simulink model "Task12"  (R2022b)
settings: Solver=VariableStepAuto  StartTime=0.0  StopTime=10.0  RelTol=1e-3
settings Model: Creator=LOQ  LastModifiedBy=LOQ
settings OptimizationCC: ReuseModelBlockBuffer=on
settings RTWCC: GPUComputeCapability=5.0
settings ConfigComp: CovBoundaryAbsTol=1.0e-5

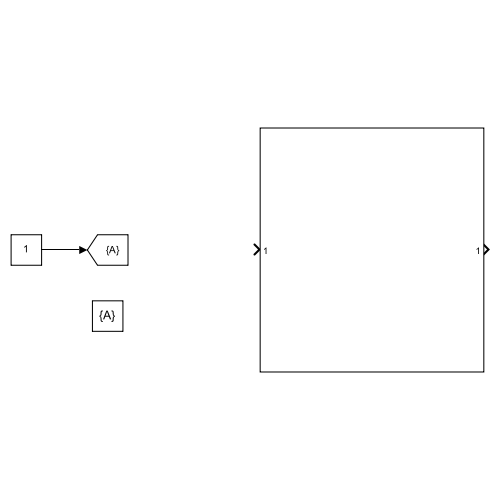
[thumbnail: Simulink's stored preview of the top-level diagram]
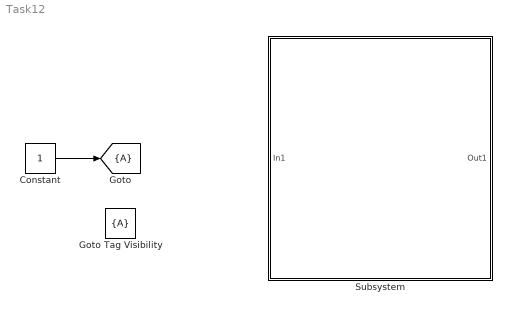
== system Task12 ==
  Constant : Constant
  Goto : Goto  TagVisibility=scoped
  Goto Tag Visibility : GotoTagVisibility
  Subsystem : Subsystem
  wires:
  Constant/1 -> Goto/1

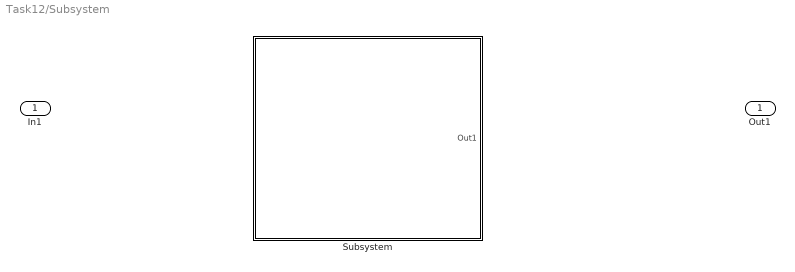
== system Task12/Subsystem ==
  In1 : Inport
  Subsystem : Subsystem
  Out1 : Outport

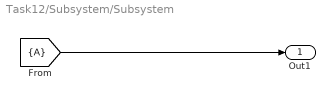
== system Task12/Subsystem/Subsystem ==
  From : From  TagVisibility=scoped
  Out1 : Outport
  wires:
  From/1 -> Out1/1
